simulink model "SeriesDCMotor"  (R2014b)
settings: Solver=ode45  StartTime=0.0  StopTime=1  MaxStep=1e-3  RelTol=1e-4  AbsTol=1e-4
values from neighbouring files (symbols this model uses):
  Dm = 6.04e-6    (= 6.04e-06)    [PMDCMotorparam.m]    (also in SeriesDCMotorparam.m = 0)
  J = 2.12e-6    (= 2.12e-06)    [PMDCMotorparam.m]    (also in SeriesDCMotorparam.m = 1000)
  Laf = 0.4631    [SeriesDCMotorparam.m]
  Ra = 7    [PMDCMotorparam.m]    (also in SeriesDCMotorparam.m = 2)
  Rf = 1    [SeriesDCMotorparam.m]
  Taf = (La+Lf)/(Ra+Rf)    (= 1.16666666667)    [SeriesDCMotorparam.m]
  Tm = 3.53e-3    (= 0.00353)    [PMDCMotorparam.m]    (also in SeriesDCMotorparam.m = 514)
  Va = 6    [PMDCMotorparam.m]    (also in SeriesDCMotorparam.m = 100)
settings Model: CovSFcnEnable=on  Creator=Jurij  LastModifiedBy=Kevin
settings DataIOCC: MaxDataPoints=10000  SignalLoggingSaveFormat=ModelDataLogs  SaveOutput=off  SaveState=on  StateSaveName=x  TimeSaveName=t  SignalLoggingName=sigsOut
settings DebuggingCC: SaveWithParameterizedLinksMsg=none  UnderspecifiedInitializationDetection=Classic  MergeDetectMultiDrivingBlocksExec=none  SignalResolutionControl=TryResolveAllWithWarning  SolverPrmCheckMsg=none  MultiTaskDSMMsg=warning  MultiTaskCondExecSysMsg=none  FrameProcessingCompatibilityMsg=error
settings HardwareCC: TargetUnknown=on
settings GRTTargetCC: CombineOutputUpdateFcns=off  GRTInterface=on

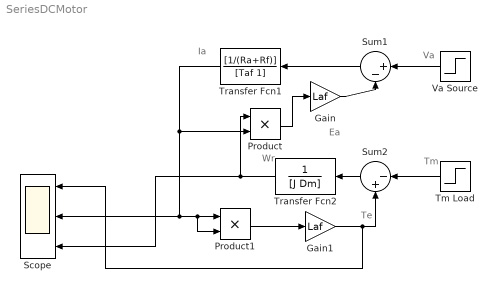
== system SeriesDCMotor ==
  note: Ia
  note: Ea
  note: Wr
  note: Te
  note: Tm
  note: Va
  Gain : Gain  Gain=Laf
  Gain1 : Gain  Gain=Laf
  Product : Product
  Product1 : Product
  Scope : Scope  NumInputPorts=3
      settings: TimeRange=1  YMin=-1~0~-50  YMax=1~0.8~250
  Sum1 : Sum  Inputs=|+-  SaturateOnIntegerOverflow=on
  Sum2 : Sum  Inputs=|-+  SaturateOnIntegerOverflow=on
  Tm Load : Step  Time=0.5  After=Tm  SampleTime=0
  Transfer Fcn1 : TransferFcn  Numerator=[1/(Ra+Rf)]  Denominator=[Taf 1]
  Transfer Fcn2 : TransferFcn  Denominator=[J Dm]
  Va Source : Step  Time=0  After=Va  SampleTime=0
  wires:
  Sum1/1 -> Transfer Fcn1/1
  Va Source/1 -> Sum1/1
  Transfer Fcn2/1 -> Product/1, Scope/3
  Product/1 -> Gain/1
  Sum2/1 -> Transfer Fcn2/1
  Tm Load/1 -> Sum2/1
  Transfer Fcn1/1 -> Product/2, Product1/2, Product1/1, Scope/2
  Product1/1 -> Gain1/1
  Gain/1 -> Sum1/2
  Gain1/1 -> Scope/1, Sum2/2
